simulink model "ta6_jointcontrol"  (R2017a)
settings: Solver=VariableStepAuto  StartTime=0.0  StopTime=10.0  RelTol=1e-3
values from neighbouring files (symbols this model uses):
  ta6 = SerialLink(L, 'name', 'hedong TA6 »úÆ÷ÈË')    [mdl_ta6.m]    (also in mdl_ta6nofri.m = SerialLink(L, 'name', 'hedong TA6 robot'))
libraries: roblocks x4
settings Model: Creator=Administrator  LastModifiedBy=Administrator

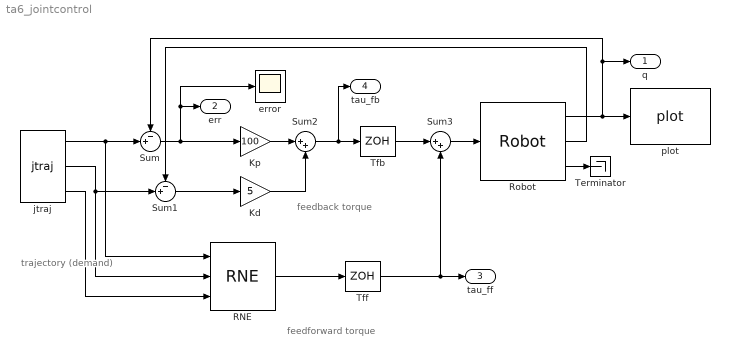
== system ta6_jointcontrol ==
  note: feedback torque
  note: trajectory
      | (demand)
  note: feedforward torque
  Kd : Gain  Gain=5  SaturateOnIntegerOverflow=on  OutDataTypeStr=Inherit: Same as input  ParamDataTypeStr=Inherit: Same as input
  Kp : Gain  Gain=100  SaturateOnIntegerOverflow=on  OutDataTypeStr=Inherit: Same as input  ParamDataTypeStr=Inherit: Same as input
  RNE : roblocks/Arm/RNE  robot=ta6.nofriction()  grav=[0 0 9.81]
  Robot : roblocks/Arm/Robot  robot=ta6.nofriction  q0=[0 0 0 0 0 0]
  Sum : Sum  Inputs=-+|  SaturateOnIntegerOverflow=on  InputSameDT=on  OutDataTypeStr=Inherit: Same as first input
  Sum1 : Sum  Inputs=-+|  SaturateOnIntegerOverflow=on  InputSameDT=on  OutDataTypeStr=Inherit: Same as first input
  Sum2 : Sum  Inputs=|++  SaturateOnIntegerOverflow=on  InputSameDT=on  OutDataTypeStr=Inherit: Same as first input
  Sum3 : Sum  Inputs=|++  SaturateOnIntegerOverflow=on  InputSameDT=on  OutDataTypeStr=Inherit: Same as first input
  Terminator : Terminator
  Tfb : ZeroOrderHold  SampleTime=0.002
  Tff : ZeroOrderHold  SampleTime=0.05
  error : Scope
  jtraj : roblocks/Toolbox/jtraj  q0=[0 0 0 0 0 0]  qf=[pi/4 pi/2 -pi/2 0 0 0]  tmax=5  ts=0.02
  plot : roblocks/Arm/plot  robot=ta6  fps=10  holdplot=on
  q : Outport
  err : Outport  Port=2
  tau_ff : Outport  Port=3
  tau_fb : Outport  Port=4
  wires:
  Robot/3 -> Terminator/1
  jtraj/2 -> Sum1/2, RNE/2
  jtraj/3 -> RNE/3
  Tff/1 -> Sum3/2, tau_ff/1
  Sum1/1 -> Kd/1
  jtraj/1 -> RNE/1, Sum/2
  Robot/1 -> Sum/1, q/1, plot/1
  Sum2/1 -> Tfb/1, tau_fb/1
  Robot/2 -> Sum1/1
  RNE/1 -> Tff/1
  Kp/1 -> Sum2/1
  Tfb/1 -> Sum3/1
  Sum3/1 -> Robot/1
  Sum/1 -> error/1, err/1, Kp/1
  Kd/1 -> Sum2/2
